simulink model "Stinger"  (R2020a)
settings: Solver=ode15s  StartTime=0.0  StopTime=10  RelTol=1e-3  EnableMultiTasking=on
undefined symbols (not defined in the file): a, Fuselage, J, Ke, kt, kv, LeftAftArm, LeftAftBall, LeftAftProp, LeftAftSkid, LeftArm, LeftArms, LeftFrontArm, LeftFrontBall, LeftFrontProp, LeftFrontSkid, LeftProp, LeftSkids, R, RightAftArm, RightAftBall, RightAftProp, RightAftSkid, RightArm, RightArms, RightFrontArm, RightFrontBall, RightFrontProp, RightFrontSkid, RightProp, RightSkids, sigbuilder_block, w0, X, Y, Z
libraries: sm_lib x167, nesl_utility x70
(part 1 of 4)
settings Model: Creator=G_MAMAN  LastModifiedBy=G_MAMAN
settings DataIOCC: LimitDataPoints=on  MaxDataPoints=10000
settings OptimizationCC: LifeSpan=inf
settings DebuggingCC: AllowSymbolicDim=off  SFUnexpectedBacktrackingDiag=warning  SFNoUnconditionalDefaultTransitionDiag=warning  SFExecutionAtInitializationDiag=none  ArithmeticOperatorsInVariantConditions=warning
settings SFSimCC: SimUseLocalCustomCode=off  CustomCodeUndefinedFunction=UseInterfaceOnly
settings RTWCC: RTWUseLocalCustomCode=off
settings CodeAppCC: StateflowObjectComments=on
settings GRTTargetCC: TargetLangStandard=C89/C90 (ANSI)
settings ConfigComp: CovMetricSettings=dw  CovHtmlReporting=on  CovSaveCumulativeToWorkspaceVar=on  CovSaveSingleToWorkspaceVar=on  CovExternalEMLEnable=off  CovSFcnEnable=off
settings SimscapeCC: SimscapeLogType=all  SimscapeLogSimulationStatistics=on  SimscapeLogDataHistory=10000
settings DiagnosticsConfigSet: SimMechanicsRigidlyBoundBlock=none

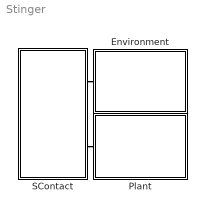
== system Stinger ==
  Environment : Subsystem  mask{E=15, P=1, Z=0.105, K=5, BIG=5}
      mask prompts: E "Size of Ground (m)"; P "Height of Ground (m)"; Z "Displacement of Ground (m)"; K "Distance Between Clouds (m)"; BIG "Size of Sun (m)"
      mask Display: image('environment.jpg'); % Use "Edit Image" on toolstrip to change.
  Plant : Subsystem  mask{s=6, g=9.80665}
      mask prompts: s "Shape (# Sides)"; g "Gravitational Acceleration (m/s^2)"
      mask Display: image('plant.png'); % Use "Edit Image" on toolstrip to change.
  SContact : Subsystem  mask{st=4e5, b=4e4, trans=1e-4, mus=0.9, mud=0.8, vcr=1e-1}
      mask prompts: st "Stiffness (N/m)"; b "Damping (N/(m/s))"; trans "Transition Region Width (m)"; mus "Coefficient of Static Friction"; mud "Coefficient of Dynamic Friction"; vcr "Critical Velocity (m/s)"
      mask Display: image('contact.jpg'); % Use "Edit Image" on toolstrip to change.
  connections:
  SContact/RConn1 -- Environment/LConn1
  SContact/RConn2 -- Plant/RConn1

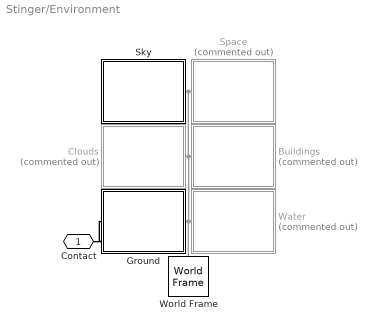
== system Stinger/Environment ==
  Buildings : Subsystem  Commented=on  mask{rhoB=1000, rgbB=[0.58 0.23 0.19], opB=1}
      mask prompts: rhoB "Density of Buildings (kg/m^3)"; rgbB "Color of Buildings [R G B]"; opB "Opacity of Buildings (0-1)"
      mask Display: image('buildings.jpg'); % Use "Edit Image" on toolstrip to change.
  Clouds : Subsystem  Commented=on  mask{rhoC=0.01, rgbC=[1 1 1], opC=0.8}
      mask prompts: rhoC "Density of Clouds (kg/m^3)"; rgbC "Color of Clouds [R G B]"; opC "Opacity of Clouds (0-1)"
      mask Display: image('clouds.jpg'); % Use "Edit Image" on toolstrip to change.
  Ground : Subsystem  mask{rhoE=1000000, rgbE=[0.609375 0.68359375 0.53125], opE=1}
      mask prompts: rhoE "Density of Ground (kg/m^3)"; rgbE "Color of Ground [R G B]"; opE "Opacity of Ground (0-1)"
      mask Display: image('ground.jpg'); % Use "Edit Image" on toolstrip to change.
  Sky : Subsystem  mask{rhoS=0.000001, rgbS=[0.529 0.808 0.922], opS=0.5}
      mask prompts: rhoS "Density of Sky (kg/m^3)"; rgbS "Color of Sky [R G B]"; opS "Opacity of Sky (0-1)"
      mask Display: image('sky.jpg'); % Use "Edit Image" on toolstrip to change.
  Space : Subsystem  Commented=on  mask{rhoN=10000000000000000, rgbN=[1 1 0], opN=0.5, rhoM=1000000, rgbM=[1 1 1], opM=0.4}
      mask prompts: rhoN "Density of Sun (kg/m^3)"; rgbN "Color of Sun [R G B]"; opN "Opacity of Sun (0-1)"; rhoM "Density of Moon (kg/m^3)"; rgbM "Color of Moon [R G B]"; opM "Opacity of Moon (0-1)"
      mask Display: image('space.jpg'); % Use "Edit Image" on toolstrip to change.
  Water : Subsystem  Commented=on  mask{rhoR=1, rgbR=[0.529 0.808 1], opR=1}
      mask prompts: rhoR "Density of Water (kg/m^3)"; rgbR "Color of Water [R G B]"; opR "Opacity of Water (0-1)"
      mask Display: image('water.jpg'); % Use "Edit Image" on toolstrip to change.
  World Frame : sm_lib/Frames and Transforms/World Frame
  Contact : PMIOPort  Side=Left
  connections:
  Contact/RConn1 -- Ground/LConn1
  Space/LConn1 -- Buildings/RConn1 -- Clouds/RConn1 -- Water/LConn1 -- World Frame/RConn1 -- Ground/RConn1 -- Sky/RConn1

== system Stinger/Plant ==
  Mechanism Configuration : sm_lib/Utilities/Mechanism Configuration  UniformGravity=Constant  GravityVector=[0 0 -g]  GravityUnits=m/s^2  LinearizationDelta=0.001
  Solver Configuration : nesl_utility/Solver Configuration  PhysicalDomain=network_engine_domain  SubClassName=solver  LeftPortType=input  RightPortType=generic  Tones=[]  Harmonics=[]  SimulateNoise=off  Profile=off  UseLocalSampling=off  EnableSwitchedLinearOptims=on  FrequencyDomain=off  UseCCode=off  RelTol=0.001  AbsTol=1e-06  MinStep=1e-09  ToWorkspace=off  RevertToSquareIcSolve=off  NumHomotopyIterations=100  PhasorMode=off  PhasorModeNumHarmonics=1  DoDC=off  ResidualTolerance=1e-09  UseLocalSolver=off  LocalSolverChoice=NE_BACKWARD_EULER_ADVANCER  LocalSolverSampleTime=0.001  DoFixedCost=off  MaxNonlinIter=3  MaxModeIter=2  LinearAlgebra=auto  EquationFormulation=NE_TIME_EF  DelaysMemoryBudget=1024  AutomaticFiltering=on  FilteringTimeConstant=0.001  PartitionStorageMethod=AS_NEEDED  PartitionMemoryBudget=1024  PartitionMethod=ROBUST
  UAV : Subsystem  mask{D=0.235, H=0.051, rho=1240, rgb=[0 0 0], op=1}
      mask prompts: D "Length of Fuselage (m)"; H "Height of Fuselage (m)"; rho "Density of Fuselage (kg/m^3)"; rgb "Color of Fuselage [R G B]"; op "Opacity of Fuselage (0-1)"
      mask Display: image('uavpic.png'); % Use "Edit Image" on toolstrip to change.
  Contact : PMIOPort  Side=Right
  connections:
  Mechanism Configuration/RConn1 -- UAV/RConn2 -- Solver Configuration/RConn1 -- UAV/RConn1
  UAV/RConn3 -- Contact/RConn1

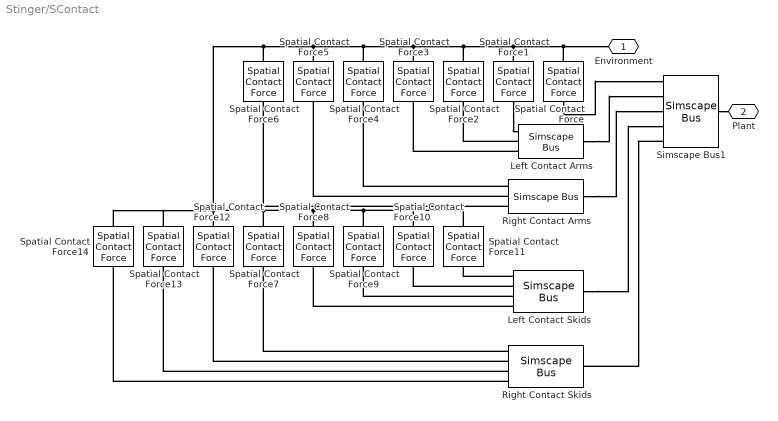
== system Stinger/SContact ==
  Left Contact Arms : SimscapeBus  HierarchyStrings=LeftFrontArm;LeftArm;LeftAftArm
  Left Contact Skids : SimscapeBus  HierarchyStrings=LeftFrontSkid;LeftFrontBall;LeftAftBall;LeftAftSkid
  Right Contact Arms : SimscapeBus  HierarchyStrings=RightFrontArm;RightArm;RightAftArm
  Right Contact Skids : SimscapeBus  HierarchyStrings=RightFrontSkid;RightFrontBall;RightAftBall;RightAftSkid
  Simscape Bus1 : SimscapeBus  HierarchyStrings=Fuselage;LeftArms;RightArms;LeftSkids;RightSkids
  Spatial Contact Force{,1..14} (15 alike) : sm_lib/Forces and Torques/Spatial Contact Force  CoefficientOfDynamicFriction=mud  CoefficientOfStaticFriction=mus  NormalDamping=b  NormalDampingUnits=N/(m/s)  NormalStiffness=st  NormalStiffnessUnits=N/m  FrictionalCriticalVelocity=vcr  FrictionalCriticalVelocityUnits=m/s  ZeroCrossDetectContactStartAndEnd=off  SenseFrictionalForceMagnitude=off  SenseNormalForceMagnitude=off  SenseSeparationDistance=off  NormalTransitionRegionWidth=trans  NormalTransitionRegionWidthUnits=m  FrictionType=SmoothStickSlip
  Environment : PMIOPort  Side=Right
  Plant : PMIOPort  Port=2  Side=Right
  connections:
  Spatial Contact Force/RConn1 -- Environment/RConn1 -- Spatial Contact Force7/RConn1 -- Spatial Contact Force8/RConn1 -- Spatial Contact Force9/RConn1 -- Spatial Contact Force10/RConn1 -- Spatial Contact Force11/RConn1 -- Spatial Contact Force12/RConn1 -- Spatial Contact Force13/RConn1 -- Spatial Contact Force14/RConn1 -- Spatial Contact Force6/RConn1 -- Spatial Contact Force5/RConn1 -- Spatial Contact Force4/RConn1 -- Spatial Contact Force3/RConn1 -- Spatial Contact Force2/RConn1 -- Spatial Contact Force1/RConn1
  Right Contact Arms/LConn3 -- Spatial Contact Force6/LConn1
  Right Contact Arms/LConn2 -- Spatial Contact Force5/LConn1
  Right Contact Skids/LConn2 -- Spatial Contact Force12/LConn1
  Left Contact Skids/LConn4 -- Spatial Contact Force8/LConn1
  Simscape Bus1/LConn5 -- Right Contact Skids/RConn1
  Right Contact Arms/LConn1 -- Spatial Contact Force4/LConn1
  Left Contact Skids/RConn1 -- Simscape Bus1/LConn4
  Left Contact Arms/LConn2 -- Spatial Contact Force2/LConn1
  Spatial Contact Force/LConn1 -- Simscape Bus1/LConn1
  Simscape Bus1/RConn1 -- Plant/RConn1
  Spatial Contact Force1/LConn1 -- Left Contact Arms/LConn1
  Left Contact Arms/RConn1 -- Simscape Bus1/LConn2
  Left Contact Skids/LConn1 -- Spatial Contact Force11/LConn1
  Right Contact Skids/LConn1 -- Spatial Contact Force7/LConn1
  Left Contact Arms/LConn3 -- Spatial Contact Force3/LConn1
  Right Contact Arms/RConn1 -- Simscape Bus1/LConn3
  Left Contact Skids/LConn2 -- Spatial Contact Force10/LConn1
  Right Contact Skids/LConn3 -- Spatial Contact Force13/LConn1
  Right Contact Skids/LConn4 -- Spatial Contact Force14/LConn1
  Left Contact Skids/LConn3 -- Spatial Contact Force9/LConn1

== system Stinger/Environment/Buildings ==
  Building 1 : sm_lib/Body Elements/Brick Solid  GraphicAmbientColor=[0.15 0.15 0.15 1.0]  BasedOnType=Density  BrickDimensions=[1 1 1]  BrickDimensionUnits=m  CenterOfMass=[0 0 0]  CenterOfMassUnits=m  GraphicDiffuseColor=rgbB  Density=rhoB  DensityUnits=kg/m^3  DoExposeReferenceFrame=on  GraphicEmissiveColor=[0.0 0.0 0.0 1.0]  ExportEntireGeometry=off  SerializedFrames=<Frames/>  MarkerShape=Sphere  MarkerSize=10  GraphicType=FromGeometry  InertiaType=CalculateFromGeometry  Mass=1  MassUnits=kg  MomentsOfInertia=[1 1 1]  MomentsOfInertiaUnits=kg*m^2  GraphicOpacity=opB  ProductsOfInertia=[0 0 0]  ProductsOfInertiaUnits=kg*m^2  GraphicShininess=75  GraphicSpecularColor=[0.5 0.5 0.5 1.0]  GraphicVisPropType=SimpleVisualProperties
  Rigid Transform : sm_lib/Frames and Transforms/Rigid Transform  TranslationMethod=None  TranslationStandardOffset=0  TranslationLengthUnit=m  TranslationStandardAxis=+Z  TranslationCartesianOffset=[0 0 0]  TranslationROffset=0  TranslationROffsetUnits=m  TranslationZOffset=0  TranslationZOffsetUnits=m  TranslationThetaOffset=0  TranslationThetaOffsetUnits=deg  RotationMethod=None  RotationAngleUnits=deg  RotationStandardAxis=+Z  RotationAngle=0.0  RotationArbitraryAxis=[0 0 1]  FollAlignAxisA=+X  BaseAlignAxisA=+Y  FollAlignAxisB=+Y  BaseAlignAxisB=+Z  RotationSequenceAxes=FollowerAxes  RotationSequence=XYX  RotationSequenceAngles=[0 0 0]  RotationSequenceAnglesUnits=deg  RotationMatrix=[1 0 0; 0 1 0; 0 0 1]
  Buildings : PMIOPort  Side=Right
  connections:
  Rigid Transform/RConn1 -- Buildings/RConn1
  Rigid Transform/LConn1 -- Building 1/RConn1

== system Stinger/Environment/Clouds ==
  Clouds1 : sm_lib/Body Elements/File Solid  ExtGeomFileName=C:\Users\G_MAMAN\Downloads\cloud.CATPart  UnitType=FromFile  ExtGeomFileUnits=m  StepReaderType=HEX  ExportConvexHullGeometry=off  InertiaType=CalculateFromGeometry  Mass=1  MassUnits=kg  CenterOfMass=[0 0 0]  CenterOfMassUnits=m  MomentsOfInertia=[1 1 1]  MomentsOfInertiaUnits=kg*m^2  ProductsOfInertia=[0 0 0]  ProductsOfInertiaUnits=kg*m^2  BasedOnType=Density  Density=rhoC  DensityUnits=kg/m^3  DoExposeReferenceFrame=on  SerializedFrames=<Frames/>  GraphicType=FromGeometry  MarkerShape=Sphere  MarkerSize=10  GraphicVisPropType=SimpleVisualProperties  GraphicDiffuseColor=rgbC  GraphicSpecularColor=[0.5 0.5 0.5 1.0]  GraphicAmbientColor=[0.15 0.15 0.15 1.0]  GraphicEmissiveColor=[0.0 0.0 0.0 1.0]  GraphicShininess=75  GraphicOpacity=opC
  Clouds2 : sm_lib/Body Elements/File Solid  ExtGeomFileName=C:\Users\G_MAMAN\Downloads\cloud.CATPart  UnitType=FromFile  ExtGeomFileUnits=m  StepReaderType=HEX  ExportConvexHullGeometry=off  InertiaType=CalculateFromGeometry  Mass=1  MassUnits=kg  CenterOfMass=[0 0 0]  CenterOfMassUnits=m  MomentsOfInertia=[1 1 1]  MomentsOfInertiaUnits=kg*m^2  ProductsOfInertia=[0 0 0]  ProductsOfInertiaUnits=kg*m^2  BasedOnType=Density  Density=rhoC  DensityUnits=kg/m^3  DoExposeReferenceFrame=on  SerializedFrames=<Frames/>  GraphicType=FromGeometry  MarkerShape=Sphere  MarkerSize=10  GraphicVisPropType=SimpleVisualProperties  GraphicDiffuseColor=rgbC  GraphicSpecularColor=[0.5 0.5 0.5 1.0]  GraphicAmbientColor=[0.15 0.15 0.15 1.0]  GraphicEmissiveColor=[0.0 0.0 0.0 1.0]  GraphicShininess=75  GraphicOpacity=opC
  Displacement3 : sm_lib/Frames and Transforms/Rigid Transform  TranslationMethod=Cartesian  TranslationStandardOffset=E/2  TranslationLengthUnit=m  TranslationStandardAxis=+Z  TranslationCartesianOffset=[50 -E/2+P 0]  TranslationROffset=0  TranslationROffsetUnits=m  TranslationZOffset=0  TranslationZOffsetUnits=m  TranslationThetaOffset=0  TranslationThetaOffsetUnits=deg  RotationMethod=StandardAxis  RotationAngleUnits=deg  RotationStandardAxis=-Y  RotationAngle=90  RotationArbitraryAxis=[0 0 1]  FollAlignAxisA=+X  BaseAlignAxisA=+Y  FollAlignAxisB=+Y  BaseAlignAxisB=+Z  RotationSequenceAxes=FollowerAxes  RotationSequence=XYX  RotationSequenceAngles=[0 0 0]  RotationSequenceAnglesUnits=deg  RotationMatrix=[1 0 0; 0 1 0; 0 0 1]
  Distance Constraint : sm_lib/Constraints/Distance Constraint  Distance=K  DistanceUnits=m  SenseSignedForceMagnitude=off  SenseTorque=off  SenseForce=off  WrenchDir=FollowerOnBase  WrenchFrame=BaseFrame
      settings: SourceProductBaseCode=MS
  Clouds : PMIOPort  Side=Right
  connections:
  Distance Constraint/RConn1 -- Clouds1/RConn1
  Displacement3/RConn1 -- Clouds/RConn1
  Displacement3/LConn1 -- Distance Constraint/LConn1 -- Clouds2/RConn1

== system Stinger/Environment/Ground ==
  Displacement : sm_lib/Frames and Transforms/Rigid Transform  TranslationMethod=StandardAxis  TranslationStandardOffset=P/2+Z  TranslationLengthUnit=m  TranslationStandardAxis=+Z  TranslationCartesianOffset=[0 0 0]  TranslationROffset=0  TranslationROffsetUnits=m  TranslationZOffset=0  TranslationZOffsetUnits=m  TranslationThetaOffset=0  TranslationThetaOffsetUnits=deg  RotationMethod=None  RotationAngleUnits=deg  RotationStandardAxis=+X  RotationAngle=90  RotationArbitraryAxis=[0 0 1]  FollAlignAxisA=+X  BaseAlignAxisA=+Y  FollAlignAxisB=+Y  BaseAlignAxisB=+Z  RotationSequenceAxes=FollowerAxes  RotationSequence=XYX  RotationSequenceAngles=[0 0 0]  RotationSequenceAnglesUnits=deg  RotationMatrix=[1 0 0; 0 1 0; 0 0 1]
  Earth : sm_lib/Body Elements/Brick Solid  GraphicAmbientColor=[0.15 0.15 0.15 1.0]  BasedOnType=Density  BrickDimensions=[E E P]  BrickDimensionUnits=m  CenterOfMass=[0 0 0]  CenterOfMassUnits=m  GraphicDiffuseColor=rgbE  Density=rhoE  DensityUnits=kg/m^3  DoExposeReferenceFrame=on  GraphicEmissiveColor=[0.0 0.0 0.0 1.0]  ExportEntireGeometry=on  SerializedFrames=<Frames/>  MarkerShape=Sphere  MarkerSize=10  GraphicType=FromGeometry  InertiaType=CalculateFromGeometry  Mass=1  MassUnits=kg  MomentsOfInertia=[1 1 1]  MomentsOfInertiaUnits=kg*m^2  GraphicOpacity=opE  ProductsOfInertia=[0 0 0]  ProductsOfInertiaUnits=kg*m^2  GraphicShininess=75  GraphicSpecularColor=[0.5 0.5 0.5 1.0]  GraphicVisPropType=SimpleVisualProperties
  Contact : PMIOPort  Side=Left
  Ground : PMIOPort  Port=2  Side=Right
  connections:
  Earth/RConn1 -- Displacement/LConn1
  Contact/RConn1 -- Earth/LConn1
  Ground/RConn1 -- Displacement/RConn1

== system Stinger/Environment/Sky ==
  Aft Sky : sm_lib/Body Elements/Brick Solid  GraphicAmbientColor=[0.15 0.15 0.15 1.0]  BasedOnType=Density  BrickDimensions=[E E P]  BrickDimensionUnits=m  CenterOfMass=[0 0 0]  CenterOfMassUnits=m  GraphicDiffuseColor=rgbS  Density=rhoS  DensityUnits=kg/m^3  DoExposeReferenceFrame=on  GraphicEmissiveColor=[0.0 0.0 0.0 1.0]  ExportEntireGeometry=off  SerializedFrames=<Frames/>  MarkerShape=Sphere  MarkerSize=10  GraphicType=FromGeometry  InertiaType=CalculateFromGeometry  Mass=1  MassUnits=kg  MomentsOfInertia=[1 1 1]  MomentsOfInertiaUnits=kg*m^2  GraphicOpacity=opS  ProductsOfInertia=[0 0 0]  ProductsOfInertiaUnits=kg*m^2  GraphicShininess=75  GraphicSpecularColor=[0.5 0.5 0.5 1.0]  GraphicVisPropType=SimpleVisualProperties
  Displacement1 : sm_lib/Frames and Transforms/Rigid Transform  TranslationMethod=Cartesian  TranslationStandardOffset=E/2  TranslationLengthUnit=m  TranslationStandardAxis=+Z  TranslationCartesianOffset=[0 -E/2+Z+P E/2+P/2]  TranslationROffset=0  TranslationROffsetUnits=m  TranslationZOffset=0  TranslationZOffsetUnits=m  TranslationThetaOffset=0  TranslationThetaOffsetUnits=deg  RotationMethod=None  RotationAngleUnits=deg  RotationStandardAxis=+X  RotationAngle=90  RotationArbitraryAxis=[0 0 1]  FollAlignAxisA=+X  BaseAlignAxisA=+Y  FollAlignAxisB=+Y  BaseAlignAxisB=+Z  RotationSequenceAxes=FollowerAxes  RotationSequence=XYX  RotationSequenceAngles=[0 0 0]  RotationSequenceAnglesUnits=deg  RotationMatrix=[1 0 0; 0 1 0; 0 0 1]
  Displacement2 : sm_lib/Frames and Transforms/Rigid Transform  TranslationMethod=None  TranslationStandardOffset=Z  TranslationLengthUnit=m  TranslationStandardAxis=+Z  TranslationCartesianOffset=[0 0 0]  TranslationROffset=0  TranslationROffsetUnits=m  TranslationZOffset=0  TranslationZOffsetUnits=m  TranslationThetaOffset=0  TranslationThetaOffsetUnits=deg  RotationMethod=StandardAxis  RotationAngleUnits=deg  RotationStandardAxis=-X  RotationAngle=90  RotationArbitraryAxis=[0 0 1]  FollAlignAxisA=+X  BaseAlignAxisA=+Y  FollAlignAxisB=+Y  BaseAlignAxisB=+Z  RotationSequenceAxes=FollowerAxes  RotationSequence=XYX  RotationSequenceAngles=[0 0 0]  RotationSequenceAnglesUnits=deg  RotationMatrix=[1 0 0; 0 1 0; 0 0 1]
  Displacement6 : sm_lib/Frames and Transforms/Rigid Transform  TranslationMethod=Cartesian  TranslationStandardOffset=E/2  TranslationLengthUnit=m  TranslationStandardAxis=+Z  TranslationCartesianOffset=[E/2-Z-P 0 E/2+P/2]  TranslationROffset=0  TranslationROffsetUnits=m  TranslationZOffset=0  TranslationZOffsetUnits=m  TranslationThetaOffset=0  TranslationThetaOffsetUnits=deg  RotationMethod=None  RotationAngleUnits=deg  RotationStandardAxis=+X  RotationAngle=90  RotationArbitraryAxis=[0 0 1]  FollAlignAxisA=+X  BaseAlignAxisA=+Y  FollAlignAxisB=+Y  BaseAlignAxisB=+Z  RotationSequenceAxes=FollowerAxes  RotationSequence=XYX  RotationSequenceAngles=[0 0 0]  RotationSequenceAnglesUnits=deg  RotationMatrix=[1 0 0; 0 1 0; 0 0 1]
  Displacement7 : sm_lib/Frames and Transforms/Rigid Transform  TranslationMethod=None  TranslationStandardOffset=Z  TranslationLengthUnit=m  TranslationStandardAxis=+Z  TranslationCartesianOffset=[0 0 0]  TranslationROffset=0  TranslationROffsetUnits=m  TranslationZOffset=0  TranslationZOffsetUnits=m  TranslationThetaOffset=0  TranslationThetaOffsetUnits=deg  RotationMethod=StandardAxis  RotationAngleUnits=deg  RotationStandardAxis=-Y  RotationAngle=90  RotationArbitraryAxis=[0 0 1]  FollAlignAxisA=+X  BaseAlignAxisA=+Y  FollAlignAxisB=+Y  BaseAlignAxisB=+Z  RotationSequenceAxes=FollowerAxes  RotationSequence=XYX  RotationSequenceAngles=[0 0 0]  RotationSequenceAnglesUnits=deg  RotationMatrix=[1 0 0; 0 1 0; 0 0 1]
  Left Sky : sm_lib/Body Elements/Brick Solid  GraphicAmbientColor=[0.15 0.15 0.15 1.0]  BasedOnType=Density  BrickDimensions=[E E P]  BrickDimensionUnits=m  CenterOfMass=[0 0 0]  CenterOfMassUnits=m  GraphicDiffuseColor=rgbS  Density=rhoS  DensityUnits=kg/m^3  DoExposeReferenceFrame=on  GraphicEmissiveColor=[0.0 0.0 0.0 1.0]  ExportEntireGeometry=off  SerializedFrames=<Frames/>  MarkerShape=Sphere  MarkerSize=10  GraphicType=FromGeometry  InertiaType=CalculateFromGeometry  Mass=1  MassUnits=kg  MomentsOfInertia=[1 1 1]  MomentsOfInertiaUnits=kg*m^2  GraphicOpacity=opS  ProductsOfInertia=[0 0 0]  ProductsOfInertiaUnits=kg*m^2  GraphicShininess=75  GraphicSpecularColor=[0.5 0.5 0.5 1.0]  GraphicVisPropType=SimpleVisualProperties
  Sky : PMIOPort  Side=Right
  connections:
  Displacement7/RConn1 -- Sky/RConn1 -- Displacement2/RConn1
  Displacement6/RConn1 -- Displacement7/LConn1
  Displacement6/LConn1 -- Left Sky/RConn1
  Displacement1/LConn1 -- Aft Sky/RConn1
  Displacement2/LConn1 -- Displacement1/RConn1

== system Stinger/Environment/Space ==
  Displacement4 : sm_lib/Frames and Transforms/Rigid Transform  TranslationMethod=Cartesian  TranslationStandardOffset=Z  TranslationLengthUnit=m  TranslationStandardAxis=+Z  TranslationCartesianOffset=[-E/1.2 -E/2 -1.2*E]  TranslationROffset=0  TranslationROffsetUnits=m  TranslationZOffset=0  TranslationZOffsetUnits=m  TranslationThetaOffset=0  TranslationThetaOffsetUnits=deg  RotationMethod=None  RotationAngleUnits=deg  RotationStandardAxis=-X  RotationAngle=90  RotationArbitraryAxis=[0 0 1]  FollAlignAxisA=+X  BaseAlignAxisA=+Y  FollAlignAxisB=+Y  BaseAlignAxisB=+Z  RotationSequenceAxes=FollowerAxes  RotationSequence=XYX  RotationSequenceAngles=[0 0 0]  RotationSequenceAnglesUnits=deg  RotationMatrix=[1 0 0; 0 1 0; 0 0 1]
  Displacement5 : sm_lib/Frames and Transforms/Rigid Transform  Commented=on  TranslationMethod=Cartesian  TranslationStandardOffset=Z  TranslationLengthUnit=m  TranslationStandardAxis=+Z  TranslationCartesianOffset=[-E/1.2 -E/2 1.2*E]  TranslationROffset=0  TranslationROffsetUnits=m  TranslationZOffset=0  TranslationZOffsetUnits=m  TranslationThetaOffset=0  TranslationThetaOffsetUnits=deg  RotationMethod=None  RotationAngleUnits=deg  RotationStandardAxis=-X  RotationAngle=90  RotationArbitraryAxis=[0 0 1]  FollAlignAxisA=+X  BaseAlignAxisA=+Y  FollAlignAxisB=+Y  BaseAlignAxisB=+Z  RotationSequenceAxes=FollowerAxes  RotationSequence=XYX  RotationSequenceAngles=[0 0 0]  RotationSequenceAnglesUnits=deg  RotationMatrix=[1 0 0; 0 1 0; 0 0 1]
  Moon : sm_lib/Body Elements/File Solid  Commented=on  ExtGeomFileName=C:\Users\G_MAMAN\Downloads\moon-rendering-1.snapshot.5\moon.SLDPRT  UnitType=Custom  ExtGeomFileUnits=m  StepReaderType=HEX  ExportConvexHullGeometry=off  InertiaType=CalculateFromGeometry  Mass=1  MassUnits=kg  CenterOfMass=[0 0 0]  CenterOfMassUnits=m  MomentsOfInertia=[1 1 1]  MomentsOfInertiaUnits=kg*m^2  ProductsOfInertia=[0 0 0]  ProductsOfInertiaUnits=kg*m^2  BasedOnType=Density  Density=rhoM  DensityUnits=kg/m^3  DoExposeReferenceFrame=on  SerializedFrames=<Frames/>  GraphicType=FromGeometry  MarkerShape=Sphere  MarkerSize=10  GraphicVisPropType=SimpleVisualProperties  GraphicDiffuseColor=rgbM  GraphicSpecularColor=[0.5 0.5 0.5 1.0]  GraphicAmbientColor=[0.15 0.15 0.15 1.0]  GraphicEmissiveColor=[0.0 0.0 0.0 1.0]  GraphicShininess=75  GraphicOpacity=opM
  Sun : sm_lib/Body Elements/Variable Mass/Variable Spherical Solid  RadiusType=Constant  Radius=BIG  RadiusUnits=m  MassType=CalculateFromGeometry  InitialMassType=Specified  InitialMass=1  InitialMassUnits=kg  Density=rhoN  DensityUnits=kg/m^3  SenseRadius=off  SenseMass=off  SenseCenterOfMass=off  SenseInertiaMatrix=off  GraphicType=FromGeometry  MarkerShape=Sphere  MarkerSize=10  GraphicVisPropType=SimpleVisualProperties  GraphicDiffuseColor=rgbN  GraphicSpecularColor=[0.5 0.5 0.5 1.0]  GraphicAmbientColor=[0.15 0.15 0.15 1.0]  GraphicEmissiveColor=[0.0 0.0 0.0 1.0]  GraphicShininess=75  GraphicOpacity=opN
      settings: SourceProductBaseCode=MS
  Space : PMIOPort  Side=Left
  connections:
  Displacement5/LConn1 -- Moon/RConn1
  Displacement4/LConn1 -- Sun/RConn1
  Displacement4/RConn1 -- Space/RConn1 -- Displacement5/RConn1

== system Stinger/Environment/Water ==
  Displacement10 : sm_lib/Frames and Transforms/Rigid Transform  TranslationMethod=Cartesian  TranslationStandardOffset=E/2  TranslationLengthUnit=m  TranslationStandardAxis=+Z  TranslationCartesianOffset=[E/2-Z-P/2 0 E/2]  TranslationROffset=0  TranslationROffsetUnits=m  TranslationZOffset=0  TranslationZOffsetUnits=m  TranslationThetaOffset=0  TranslationThetaOffsetUnits=deg  RotationMethod=None  RotationAngleUnits=deg  RotationStandardAxis=+X  RotationAngle=90  RotationArbitraryAxis=[0 0 1]  FollAlignAxisA=+X  BaseAlignAxisA=+Y  FollAlignAxisB=+Y  BaseAlignAxisB=+Z  RotationSequenceAxes=FollowerAxes  RotationSequence=XYX  RotationSequenceAngles=[0 0 0]  RotationSequenceAnglesUnits=deg  RotationMatrix=[1 0 0; 0 1 0; 0 0 1]
  Displacement11 : sm_lib/Frames and Transforms/Rigid Transform  TranslationMethod=None  TranslationStandardOffset=Z  TranslationLengthUnit=m  TranslationStandardAxis=+Z  TranslationCartesianOffset=[0 0 0]  TranslationROffset=0  TranslationROffsetUnits=m  TranslationZOffset=0  TranslationZOffsetUnits=m  TranslationThetaOffset=0  TranslationThetaOffsetUnits=deg  RotationMethod=StandardAxis  RotationAngleUnits=deg  RotationStandardAxis=-Y  RotationAngle=90  RotationArbitraryAxis=[0 0 1]  FollAlignAxisA=+X  BaseAlignAxisA=+Y  FollAlignAxisB=+Y  BaseAlignAxisB=+Z  RotationSequenceAxes=FollowerAxes  RotationSequence=XYX  RotationSequenceAngles=[0 0 0]  RotationSequenceAnglesUnits=deg  RotationMatrix=[1 0 0; 0 1 0; 0 0 1]
  Displacement8 : sm_lib/Frames and Transforms/Rigid Transform  TranslationMethod=Cartesian  TranslationStandardOffset=E/2  TranslationLengthUnit=m  TranslationStandardAxis=+Z  TranslationCartesianOffset=[E/2-Z-P/2 0 E/2]  TranslationROffset=0  TranslationROffsetUnits=m  TranslationZOffset=0  TranslationZOffsetUnits=m  TranslationThetaOffset=0  TranslationThetaOffsetUnits=deg  RotationMethod=None  RotationAngleUnits=deg  RotationStandardAxis=+X  RotationAngle=90  RotationArbitraryAxis=[0 0 1]  FollAlignAxisA=+X  BaseAlignAxisA=+Y  FollAlignAxisB=+Y  BaseAlignAxisB=+Z  RotationSequenceAxes=FollowerAxes  RotationSequence=XYX  RotationSequenceAngles=[0 0 0]  RotationSequenceAnglesUnits=deg  RotationMatrix=[1 0 0; 0 1 0; 0 0 1]
  Displacement9 : sm_lib/Frames and Transforms/Rigid Transform  TranslationMethod=Cartesian  TranslationStandardOffset=E/2  TranslationLengthUnit=m  TranslationStandardAxis=+Z  TranslationCartesianOffset=[E/2-Z-P/2 0 E/2]  TranslationROffset=0  TranslationROffsetUnits=m  TranslationZOffset=0  TranslationZOffsetUnits=m  TranslationThetaOffset=0  TranslationThetaOffsetUnits=deg  RotationMethod=None  RotationAngleUnits=deg  RotationStandardAxis=+X  RotationAngle=90  RotationArbitraryAxis=[0 0 1]  FollAlignAxisA=+X  BaseAlignAxisA=+Y  FollAlignAxisB=+Y  BaseAlignAxisB=+Z  RotationSequenceAxes=FollowerAxes  RotationSequence=XYX  RotationSequenceAngles=[0 0 0]  RotationSequenceAnglesUnits=deg  RotationMatrix=[1 0 0; 0 1 0; 0 0 1]
  River 1 : sm_lib/Body Elements/Brick Solid  GraphicAmbientColor=[0.15 0.15 0.15 1.0]  BasedOnType=Density  BrickDimensions=[E/10 E/3 P/10]  BrickDimensionUnits=m  CenterOfMass=[0 0 0]  CenterOfMassUnits=m  GraphicDiffuseColor=rgbR  Density=rhoR  DensityUnits=kg/m^3  DoExposeReferenceFrame=on  GraphicEmissiveColor=[0.0 0.0 0.0 1.0]  ExportEntireGeometry=off  SerializedFrames=<Frames/>  MarkerShape=Sphere  MarkerSize=10  GraphicType=FromGeometry  InertiaType=CalculateFromGeometry  Mass=1  MassUnits=kg  MomentsOfInertia=[1 1 1]  MomentsOfInertiaUnits=kg*m^2  GraphicOpacity=opR  ProductsOfInertia=[0 0 0]  ProductsOfInertiaUnits=kg*m^2  GraphicShininess=75  GraphicSpecularColor=[0.5 0.5 0.5 1.0]  GraphicVisPropType=SimpleVisualProperties
  River 2 : sm_lib/Body Elements/Brick Solid  GraphicAmbientColor=[0.15 0.15 0.15 1.0]  BasedOnType=Density  BrickDimensions=[E/10 E/3 P/10]  BrickDimensionUnits=m  CenterOfMass=[0 0 0]  CenterOfMassUnits=m  GraphicDiffuseColor=rgbR  Density=rhoR  DensityUnits=kg/m^3  DoExposeReferenceFrame=on  GraphicEmissiveColor=[0.0 0.0 0.0 1.0]  ExportEntireGeometry=off  SerializedFrames=<Frames/>  MarkerShape=Sphere  MarkerSize=10  GraphicType=FromGeometry  InertiaType=CalculateFromGeometry  Mass=1  MassUnits=kg  MomentsOfInertia=[1 1 1]  MomentsOfInertiaUnits=kg*m^2  GraphicOpacity=opR  ProductsOfInertia=[0 0 0]  ProductsOfInertiaUnits=kg*m^2  GraphicShininess=75  GraphicSpecularColor=[0.5 0.5 0.5 1.0]  GraphicVisPropType=SimpleVisualProperties
  River 3 : sm_lib/Body Elements/Brick Solid  GraphicAmbientColor=[0.15 0.15 0.15 1.0]  BasedOnType=Density  BrickDimensions=[E/10 E/3 P/10]  BrickDimensionUnits=m  CenterOfMass=[0 0 0]  CenterOfMassUnits=m  GraphicDiffuseColor=rgbR  Density=rhoR  DensityUnits=kg/m^3  DoExposeReferenceFrame=on  GraphicEmissiveColor=[0.0 0.0 0.0 1.0]  ExportEntireGeometry=off  SerializedFrames=<Frames/>  MarkerShape=Sphere  MarkerSize=10  GraphicType=FromGeometry  InertiaType=CalculateFromGeometry  Mass=1  MassUnits=kg  MomentsOfInertia=[1 1 1]  MomentsOfInertiaUnits=kg*m^2  GraphicOpacity=opR  ProductsOfInertia=[0 0 0]  ProductsOfInertiaUnits=kg*m^2  GraphicShininess=75  GraphicSpecularColor=[0.5 0.5 0.5 1.0]  GraphicVisPropType=SimpleVisualProperties
  Water : PMIOPort  Side=Left
  connections:
  Displacement10/RConn1 -- Displacement8/RConn1 -- Water/RConn1 -- Displacement11/RConn1
  River 2/RConn1 -- Displacement9/LConn1
  Displacement9/RConn1 -- Displacement11/LConn1
  Displacement8/LConn1 -- River 3/RConn1
  River 1/RConn1 -- Displacement10/LConn1

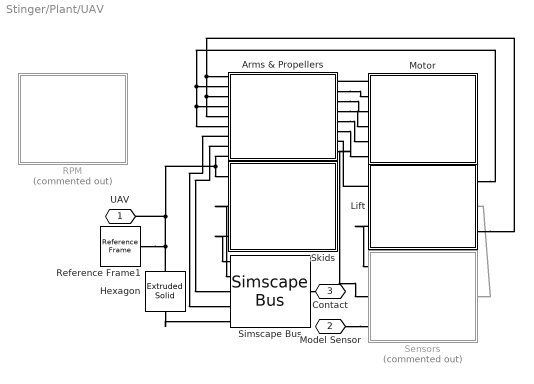
== system Stinger/Plant/UAV ==
  Arms & Propellers : Subsystem  mask{R1=0.025, L1=0.253, theta=0, Rp=0.009, Lp=0.254, rho1=1240, rhoP=1240, rgb1=[1 1 0], rgbP=[0 0 0], op1=1, opP=1}
      mask prompts: R1 "Radius of Arm (m)"; L1 "Length of Arm (m)"; theta "Arm Height Angle (deg)"; Rp "Propeller Width (m)"; Lp "Propeller Diameter (m)"; rho1 "Density of Arm (kg/m^3)"; rhoP "Density of Propeller (kg/m^3)"; rgb1 "Color of Arm [R G B]"; rgbP "Color of Propeller [R G B]"; op1 "Opacity of Arm (0-1)"; opP "Opacity of Propeller (0-1)"
      mask Display: image('armsprops.jpg'); % Use "Edit Image" on toolstrip to change.
  Hexagon : sm_lib/Body Elements/Extruded Solid  GraphicAmbientColor=[0.15 0.15 0.15 1.0]  BasedOnType=Density  CenterOfMass=[0 0 0]  CenterOfMassUnits=m  GraphicDiffuseColor=rgb  ExportConvexHullGeometry=off  ExtrusionCrossSection=[1 1; -1 1; -1 -1; 1 -1]  ExtrusionCrossSectionUnits=m  Density=rho  DensityUnits=kg/m^3  DoExposeReferenceFrame=on  GraphicEmissiveColor=[0.0 0.0 0.0 1.0]  ExportEntireGeometry=on  ExtrusionLength=H  ExtrusionLengthUnits=m  ExtrusionType=Regular  SerializedFrames=<Frames/>  MarkerShape=Sphere  MarkerSize=10  GraphicType=FromGeometry  InertiaType=CalculateFromGeometry  Mass=1  MassUnits=kg  MomentsOfInertia=[1 1 1]  MomentsOfInertiaUnits=kg*m^2  PolygonNumSides=s  GraphicOpacity=op  PolygonOuterRadius=D/2  PolygonOuterRadiusUnits=m  ProductsOfInertia=[0 0 0]  ProductsOfInertiaUnits=kg*m^2  GraphicShininess=75  GraphicSpecularColor=[0.5 0.5 0.5 1.0]  GraphicVisPropType=SimpleVisualProperties
  Lift : Subsystem  mask{F=41.7}
      mask prompts: F "Lift Force (N)"
      mask Display: image('lift.jpg'); % Use "Edit Image" on toolstrip to change.
  Motor : Subsystem  mask{T1=0.01, T2=-0.01, T3=0.01, T4=-0.01, T5=0.01, T6=-0.01}
      mask prompts: T1 "Torque of Motor 1 (Nm)"; T2 "Torque of Motor 2 (Nm)"; T3 "Torque of Motor 3 (Nm)"; T4 "Torque of Motor 4 (Nm)"; T5 "Torque of Motor 5 (Nm)"; T6 "Torque of Motor 6 (Nm)"
      mask Display: image('motor.jpg'); % Use "Edit Image" on toolstrip to change.
  RPM : Subsystem  Commented=on  mask{rpm1=0.01, rpm2=0.01, rpm3=0.01, rpm4=-0.01, rpm5=-0.01, rpm6=-0.01}
      mask prompts: rpm1 "Rotation Speed of Motor 1 (RPM)"; rpm2 "Rotation Speed of Motor 2 (RPM)"; rpm3 "Rotation Speed of Motor 3 (RPM)"; rpm4 "Rotation Speed of Motor 4 (RPM)"; rpm5 "Rotation Speed of Motor 5 (RPM)"; rpm6 "Rotation Speed of Motor 6 (RPM)"
      mask Display: image('rpm.jpg'); % Use "Edit Image" on toolstrip to change.
  Reference Frame1 : sm_lib/Frames and Transforms/Reference Frame
  Sensors : Subsystem  Commented=on  mask{Parameter1=0}
      mask Display: image('sensors.jpg'); % Use "Edit Image" on toolstrip to change.
  Simscape Bus : SimscapeBus  HierarchyStrings=RightSkids;LeftSkids;RightArms;LeftArms;Fuselage
  Skids : Subsystem  mask{R2=0.01, L2=0.1, rho2=1240, rgb2=[1 1 0], op2=1, phi=60, ksi=30}
      mask prompts: R2 "Radius of Skid (m)"; L2 "Length of Skid (m)"; rho2 "Density of Skid (kg/m^3)"; rgb2 "Color of Skid [R G B]"; op2 "Opacity of Skid (0-1)"; phi "Skid Height Angle (deg)"; ksi "Skid Rotation (deg)"
      mask Display: image('skids.jpg'); % Use "Edit Image" on toolstrip to change.
  UAV : PMIOPort  Side=Right
  Model Sensor : PMIOPort  Port=2  Side=Right
  Contact : PMIOPort  Port=3  Side=Right
  connections:
  Reference Frame1/RConn1 -- Arms & Propellers/RConn9 -- Skids/LConn1 -- UAV/RConn1 -- Hexagon/RConn1
  Simscape Bus/RConn1 -- Contact/RConn1
  Lift/LConn1 -- Arms & Propellers/LConn7
  Skids/LConn3 -- Simscape Bus/LConn1
  Skids/LConn2 -- Simscape Bus/LConn2
  Arms & Propellers/RConn8 -- Simscape Bus/LConn3
  Arms & Propellers/RConn7 -- Simscape Bus/LConn4
  Hexagon/LConn1 -- Simscape Bus/LConn5
  Model Sensor/RConn1 -- Sensors/LConn3
  Arms & Propellers/LConn8 -- Sensors/LConn2
  Sensors/RConn1 -- Lift/RConn2
  Motor/RConn1 -- Arms & Propellers/LConn1
  Arms & Propellers/LConn2 -- Motor/RConn2
  Arms & Propellers/LConn3 -- Motor/RConn3
  Arms & Propellers/LConn4 -- Motor/RConn4
  Arms & Propellers/LConn5 -- Motor/RConn5
  Arms & Propellers/LConn6 -- Motor/RConn6
  Lift/LConn2 -- Sensors/LConn1
  Lift/RConn3 -- Arms & Propellers/RConn3 -- Arms & Propellers/RConn5 -- Arms & Propellers/RConn1
  Lift/RConn1 -- Arms & Propellers/RConn6 -- Arms & Propellers/RConn4 -- Arms & Propellers/RConn2
